simulink model "rs_239_255_nonoise_integer"  (R2018b)
settings: Solver=VariableStepAuto  StartTime=0.0  StopTime=10.0  RelTol=1e-3
undefined symbols (not defined in the file): rsgenpoly
libraries: commblkcod2 x2, commsink2 x1, commrandsrc3 x1
settings Model: Creator=Tejasvi  LastModifiedBy=Tejasvi

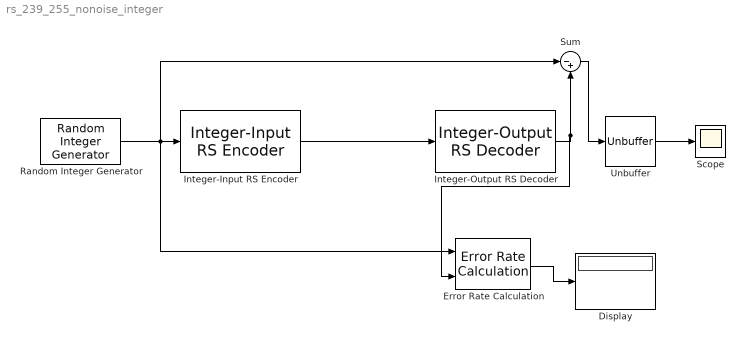
== system rs_239_255_nonoise_integer ==
  Display : Display
  Error Rate Calculation : commsink2/Error Rate Calculation  N=0  st_delay=0  cp_mode=Entire frame  subframe=[]  PMode=Port  WsName=ErrorVec  RsMode2=off  stop=off  numErr=100  maxBits=1e6
  Integer-Input RS Encoder : commblkcod2/Integer-Input RS Encoder  n=255  k=239  specShortening=off  shortenedK=3  specGenPoly=on  genPoly=rsgenpoly(255, 239, [], [], 'double')  specPrimPoly=on  prPoly='X^8 + X^4 + X^3 + X^2 + 1'  specPuncture=off  punctVec=[ones(2,1); zeros(2,1)]
      settings: SourceProductName=Communications System Toolbox  SourceProductBaseCode=CM
  Integer-Output RS Decoder : commblkcod2/Integer-Output RS Decoder  n=255  k=239  specShortening=off  shortenedK=3  specGenPoly=on  genPoly=rsgenpoly(255, 239, [], [], 'double')  specPrimPoly=on  prPoly='X^8 + X^4 + X^3 + X^2 + 1'  specPuncture=off  punctVec=[ones(2,1); zeros(2,1)]  specErasurePort=off  showNumErr=off
      settings: SourceProductName=Communications System Toolbox  SourceProductBaseCode=CM
  Random Integer Generator : commrandsrc3/Random Integer Generator  SetSize=255  SeedSource=Auto  Seed=0  SampleTime=1  SamplesPerFrame=239  OutputDataType=double  SimulateUsing=Interpreted execution
  Scope : Scope
  Sum : Sum  Inputs=|-+
  Unbuffer : Unbuffer
  wires:
  Random Integer Generator/1 -> Error Rate Calculation/1, Sum/1, Integer-Input RS Encoder/1
  Error Rate Calculation/1 -> Display/1
  Sum/1 -> Unbuffer/1
  Unbuffer/1 -> Scope/1
  Integer-Output RS Decoder/1 -> Error Rate Calculation/2, Sum/2
  Integer-Input RS Encoder/1 -> Integer-Output RS Decoder/1
